simulink model "Oshibka"  (R2017a)
settings: Solver=VariableStepAuto  StartTime=0.0  StopTime=30  MaxStep=0.101  MinStep=0.1  RelTol=1e-6
settings Model: Creator=User  LastModifiedBy=User

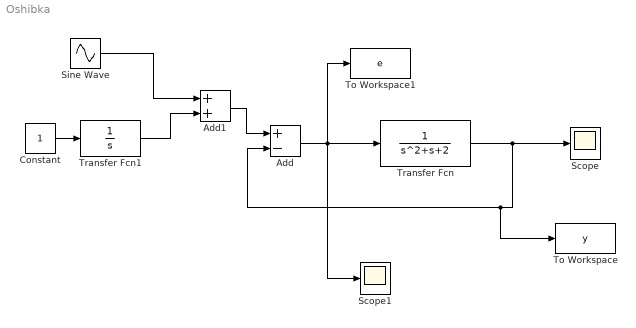
== system Oshibka ==
  Add : Sum  Inputs=+-
  Add1 : Sum
  Constant : Constant
  Scope : Scope
  Scope1 : Scope
  Sine Wave : Sin  Amplitude=0.5  Frequency=0.5  Phase=pi/2  SampleTime=0
  To Workspace : ToWorkspace  VariableName=y  SampleTime=-1
  To Workspace1 : ToWorkspace  VariableName=e  SampleTime=-1
  Transfer Fcn : TransferFcn  Denominator=[1 1 2]
  Transfer Fcn1 : TransferFcn  Denominator=[1 0]
  wires:
  Add/1 -> To Workspace1/1, Transfer Fcn/1, Scope1/1
  Transfer Fcn/1 -> To Workspace/1, Add/2, Scope/1
  Add1/1 -> Add/1
  Constant/1 -> Transfer Fcn1/1
  Transfer Fcn1/1 -> Add1/2
  Sine Wave/1 -> Add1/1
